simulink model "pendulum_model_simulink"  (R2023b)
settings: Solver=VariableStepAuto  StartTime=0.0  StopTime=endTime  MaxStep=1e-4  RelTol=1e-3
values from neighbouring files (symbols this model uses):
  alpha_0 = cutData(1)    [model_validation_data.m]    (also in pendulum_experiment.m)
  Bp_ = 1.51e-5    (= 1.51e-05)    [model_validation_data.m]    (also in pendulum_experiment.m)
  g_ = 9.81    [model_validation_data.m]    (also in pendulum_experiment.m)
  Jp_ = 2.44e-5    (= 2.44e-05)    [model_validation_data.m]    (also in pendulum_experiment.m)
  lp_ = Lp/2    (= 0.0645)    [model_validation_data.m]    (also in pendulum_experiment.m)
  mp_ = 0.024    [model_validation_data.m]    (also in pendulum_experiment.m)
settings Model: Creator=renzo  LastModifiedBy=renzo

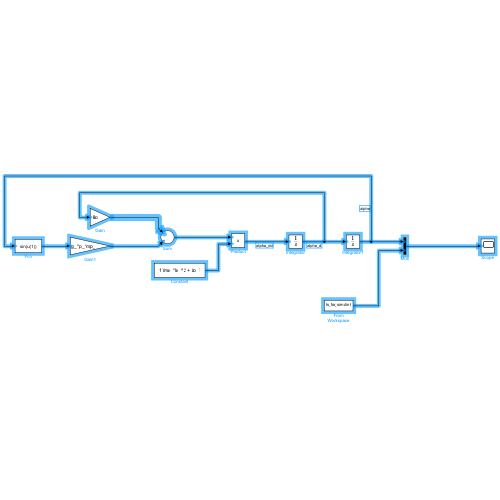
[thumbnail: Simulink's stored preview of the top-level diagram]
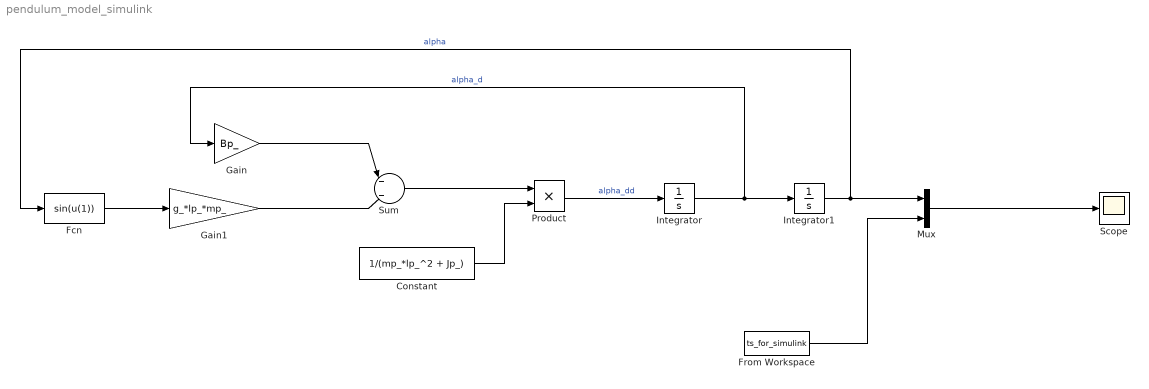
== system pendulum_model_simulink ==
  Constant : Constant  Value=1/(mp_*lp_^2 + Jp_)
  Fcn : Fcn  Expr=sin(u(1))
  From Workspace : FromWorkspace  VariableName=ts_for_simulink
  Gain : Gain  Gain=Bp_
  Gain1 : Gain  Gain=g_*lp_*mp_
  Integrator : Integrator
  Integrator1 : Integrator  InitialCondition=alpha_0
  Mux : Mux  Inputs=2
  Product : Product
  Scope : Scope
  Sum : Sum  Inputs=|-|-|
  wires:
  Mux/1 -> Scope/1
  Integrator1/1 -> Fcn/1, Mux/1  "alpha"
  Fcn/1 -> Gain1/1
  Constant/1 -> Product/2
  Product/1 -> Integrator/1  "alpha_dd"
  Gain1/1 -> Sum/2
  Integrator/1 -> Gain/1, Integrator1/1  "alpha_d"
  From Workspace/1 -> Mux/2
  Sum/1 -> Product/1
  Gain/1 -> Sum/1
